simulink model "sampleModel1796"  (R2023a)
settings: Solver=VariableStepAuto  StartTime=0.0  StopTime=10.0  RelTol=1e-3
libraries: hdlsllib x7, simulink x1
settings Model: Creator=user1  LastModifiedBy=user1

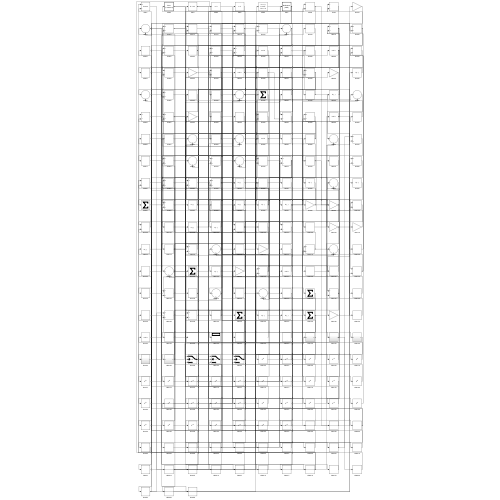
[thumbnail: Simulink's stored preview of the top-level diagram]
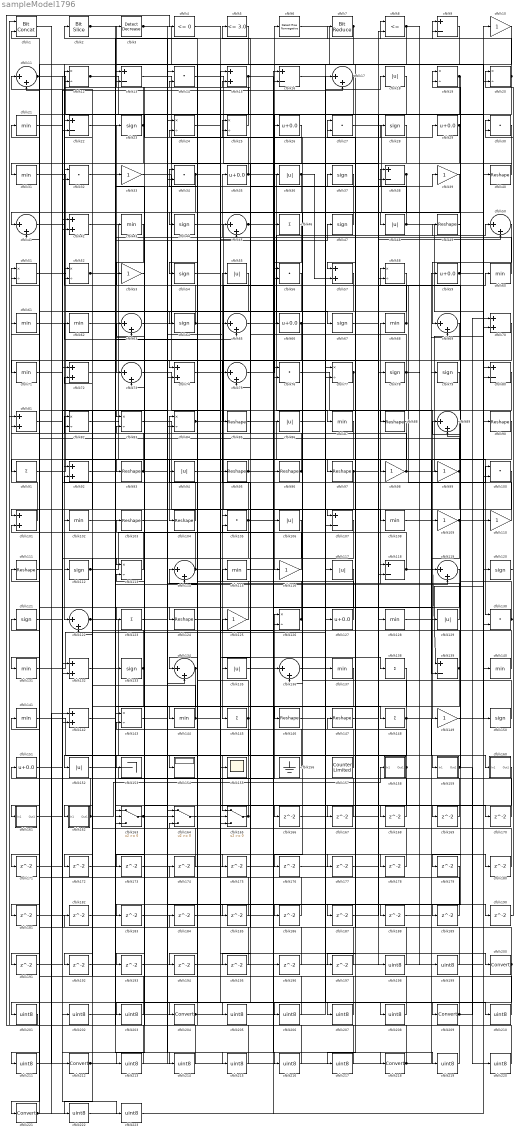
== system sampleModel1796 ==
  cfblk1 : hdlsllib/Logic and Bit Operations/Bit Concat  numInputs=2
  cfblk{10,33,39,53,98..99,109..110,116,125,149} (11 alike) : Gain
  cfblk{14,27,30,32,34,56,76,100,105,130} (10 alike) : DotProduct  OutDataTypeStr=Inherit: Inherit via internal rule
  cfblk{15,42,57,70,72,74,81,92,101,132,142} (11 alike) : Sum
  cfblk{21,31,43,60..62,68,71,87,102,108,115,128,131,137,140..141,144} (18 alike) : MinMax
  cfblk{40,49,85,88,90,93,95..97,103..104,111,124,146..147} (15 alike) : Reshape
  cfblk{18,36,48,55,86,94,106,117,129,135,152} (11 alike) : Abs  SaturateOnIntegerOverflow=off
  cfblk{9,13,16,22,38,80,107,118,139} (9 alike) : Sum  Inputs=+-
  cfblk{11,17,41,45,50,63,65,69,73,75,89,114,119,122,134,136} (16 alike) : Sum  Inputs=|++
  cfblk{23,28,37,44,47,54,64,67,78..79,112,120..121,133,150} (15 alike) : Signum
  cfblk{12,19..20,24..25,51..52,58,77,82..84,113,126,143} (15 alike) : Product  Inputs=*/  RndMeth=Zero  SaturateOnIntegerOverflow=on
  cfblk{46,91,123,138,145,148} (6 alike) : Sum  Inputs=+
  cfblk{26,29,35,59,66,127,151} (7 alike) : Bias  Bias=0.0  SaturateOnIntegerOverflow=off
  cfblk153 : Terminator
  cfblk154 : Display
  cfblk155 : Scope
  cfblk156 : Ground
  cfblk157 : hdlsllib/Sources/Counter Limited  uplimit=7  tsamp=-1
  cfblk158 : Subsystem
      settings: LibrarySourceBlock=|
      | hdlsllib/Ports &
      | Subsystems/Subsystem
  cfblk159 : Subsystem
      settings: LibrarySourceBlock=|
      | hdlsllib/Ports &
      | Subsystems/Subsystem
  cfblk160 : Subsystem
      settings: LibrarySourceBlock=|
      | hdlsllib/Ports &
      | Subsystems/Subsystem
  cfblk161 : Subsystem
      settings: LibrarySourceBlock=|
      | hdlsllib/Ports &
      | Subsystems/Subsystem
  cfblk162 : Subsystem
      settings: LibrarySourceBlock=|
      | hdlsllib/Ports &
      | Subsystems/Subsystem
  cfblk163 : Switch  SaturateOnIntegerOverflow=off  InputSameDT=off
  cfblk164 : Switch  SaturateOnIntegerOverflow=off  InputSameDT=off
  cfblk165 : Switch  SaturateOnIntegerOverflow=off  InputSameDT=off
  cfblk{166..197} (32 alike) : Delay  SampleTime=1
  cfblk{198..199,201..203,205..208,210..211,213..217,219..220,222..223} (20 alike) : DataTypeConversion  OutDataTypeStr=uint8  SaturateOnIntegerOverflow=off  RndMeth=Floor
  cfblk2 : hdlsllib/Logic and Bit Operations/Bit Slice  lidx=7  ridx=0
  cfblk{200,204,209,212,218,221} (6 alike) : DataTypeConversion  SaturateOnIntegerOverflow=off  RndMeth=Floor
  cfblk3 : simulink/Logic and Bit Operations/Detect Decrease  vinit=0.0  OutDataTypeStr=boolean
      settings: LibrarySourceBlock=|
      | hdlsllib/Logic and Bit
      | Operations/Detect
      | Decrease
  cfblk4 : hdlsllib/Logic and Bit Operations/Compare To Zero  relop=<=  OutDataTypeStr=boolean
  cfblk5 : hdlsllib/Logic and Bit Operations/Compare To Constant  relop=<=  const=3.0  OutDataTypeStr=boolean
  cfblk6 : hdlsllib/Logic and Bit Operations/Detect Rise Nonnegative  vinit=0  OutDataTypeStr=boolean
  cfblk7 : hdlsllib/Logic and Bit Operations/Bit Reduce  mode=AND
  cfblk8 : RelationalOperator  Operator=<=  OutDataTypeStr=boolean  InputSameDT=off
  wires:
  cfblk129/1 -> cfblk68/1
  cfblk63/1 -> cfblk27/1
  cfblk10/1 -> cfblk122/1
  cfblk122/1 -> cfblk154/1, cfblk47/1
  cfblk91/1 -> cfblk98/1
  cfblk68/1 -> cfblk12/1, cfblk64/1
  cfblk117/1 -> cfblk204/1
  cfblk60/1 -> cfblk35/1
  cfblk25/1 -> cfblk3/1
  cfblk152/1 -> cfblk126/1
  cfblk4/1 -> cfblk200/1
  cfblk31/1 -> cfblk93/1
  cfblk74/1 -> cfblk145/1
  cfblk87/1 -> cfblk104/1
  cfblk42/1 -> cfblk149/1
  cfblk46/1 -> cfblk116/1
  cfblk94/1 -> cfblk105/1
  cfblk64/1 -> cfblk23/1, cfblk138/1
  cfblk43/1 -> cfblk73/1
  cfblk162/1(Out1) -> cfblk158/1(In1), cfblk141/1
  cfblk66/1 -> cfblk123/1, cfblk49/1
  cfblk133/1 -> cfblk22/1, cfblk192/1
  cfblk113/1 -> cfblk103/1
  cfblk75/1 -> cfblk6/1
  cfblk56/1 -> cfblk112/1
  cfblk26/1 -> cfblk124/1
  cfblk65/1 -> cfblk50/1
  cfblk29/1 -> cfblk31/1, cfblk75/2, cfblk189/1
  cfblk17/1 -> cfblk96/1, cfblk153/1
  cfblk116/1 -> cfblk33/1
  cfblk85/1 -> cfblk130/1
  cfblk139/1 -> cfblk11/1, cfblk187/1
  cfblk130/1 -> cfblk30/1, cfblk56/2
  cfblk118/1 -> cfblk139/1, cfblk82/1
  cfblk41/1 -> cfblk52/1
  cfblk44/1 -> cfblk107/1
  cfblk47/1 -> cfblk41/1
  cfblk105/1 -> cfblk55/1, cfblk132/2, cfblk167/1
  cfblk23/1 -> cfblk101/1, cfblk12/2
  cfblk69/1 -> cfblk92/1
  cfblk28/1 -> cfblk135/1
  cfblk52/1 -> cfblk128/1, cfblk75/1
  cfblk156/1 -> cfblk115/1
  cfblk140/1 -> cfblk95/1
  cfblk83/1 -> cfblk108/1
  cfblk50/1 -> cfblk69/1
  cfblk145/1 -> cfblk152/1, cfblk114/1
  cfblk90/1 -> cfblk97/1
  cfblk34/1 -> cfblk48/1, cfblk173/1
  cfblk35/1 -> cfblk87/1, cfblk13/2
  cfblk3/1 -> cfblk137/1, cfblk186/1
  cfblk165/1 -> cfblk34/1, cfblk14/2
  cfblk134/1 -> cfblk114/2, cfblk222/1
  cfblk104/1 -> cfblk84/1
  cfblk148/1 -> cfblk165/1, cfblk160/1(In1), cfblk25/1, cfblk217/1
  cfblk7/1 -> cfblk144/1, cfblk11/2
  cfblk95/1 -> cfblk86/1, cfblk91/1
  cfblk136/1 -> cfblk18/1
  cfblk13/1 -> cfblk45/1
  cfblk125/1 -> cfblk2/1
  cfblk54/1 -> cfblk36/1
  cfblk51/1 -> cfblk67/1
  cfblk157/1 -> cfblk63/1
  cfblk30/1 -> cfblk134/1
  cfblk149/1 -> cfblk90/1
  cfblk114/1 -> cfblk29/1, cfblk51/2
  cfblk109/1 -> cfblk10/1, cfblk139/2
  cfblk84/1 -> cfblk26/1, cfblk170/1
  cfblk57/1 -> cfblk163/2
  cfblk78/1 -> cfblk43/1, cfblk99/1, cfblk146/1
  cfblk16/1 -> cfblk209/1
  cfblk98/1 -> cfblk40/1, cfblk25/2
  cfblk76/1 -> cfblk109/1
  cfblk14/1 -> cfblk78/1
  cfblk77/1 -> cfblk102/1, cfblk136/2, cfblk142/2
  cfblk49/1 -> cfblk19/1
  cfblk80/1 -> cfblk221/1
  cfblk36/1 -> cfblk57/2, cfblk193/1
  cfblk142/1 -> cfblk39/1
  cfblk27/1 -> cfblk150/1
  cfblk101/1 -> cfblk51/1
  cfblk20/1 -> cfblk107/2, cfblk9/2, cfblk191/1
  cfblk97/1 -> cfblk60/1, cfblk50/2, cfblk195/1
  cfblk8/1 -> cfblk197/1, cfblk199/1
  cfblk33/1 -> cfblk76/2
  cfblk92/1 -> cfblk133/1
  cfblk19/1 -> cfblk34/2, cfblk54/1, cfblk89/2
  cfblk121/1 -> cfblk17/2
  cfblk108/1 -> cfblk79/1
  cfblk40/1 -> cfblk32/1
  cfblk151/1 -> cfblk100/1
  cfblk22/1 -> cfblk148/1
  cfblk55/1 -> cfblk161/1(In1)
  cfblk82/1 -> cfblk119/1
  cfblk103/1 -> cfblk8/1
  cfblk110/1 -> cfblk58/1
  cfblk6/1 -> cfblk120/1
  cfblk73/1 -> cfblk155/1
  cfblk126/1 -> cfblk53/1, cfblk83/2
  cfblk141/1 -> cfblk159/1(In1)
  cfblk12/1 -> cfblk56/1, cfblk20/2
  cfblk2/1 -> cfblk119/2, cfblk208/1
  cfblk99/1 -> cfblk131/1, cfblk61/1, cfblk205/1
  cfblk61/1 -> cfblk74/1
  cfblk164/1 -> cfblk126/2
  cfblk48/1 -> cfblk70/2, cfblk5/1
  cfblk59/1 -> cfblk100/2, cfblk19/2
  cfblk93/1 -> cfblk21/1, cfblk7/1
  cfblk146/1 -> cfblk28/1
  cfblk32/1 -> cfblk164/2
  cfblk115/1 -> cfblk38/1
  cfblk143/1 -> cfblk218/1
  cfblk53/1 -> cfblk73/2
  cfblk62/1 -> cfblk9/1
  cfblk144/1 -> cfblk72/2, cfblk190/1
  cfblk11/1 -> cfblk72/1, cfblk140/1
  cfblk38/1 -> cfblk57/1, cfblk176/1
  cfblk79/1 -> cfblk88/1
  cfblk150/1 -> cfblk85/1
  cfblk5/1 -> cfblk44/1
  cfblk1/1 -> cfblk212/1
  cfblk128/1 -> cfblk110/1
  cfblk158/1(Out1) -> cfblk37/1, cfblk183/1
  cfblk21/1 -> cfblk84/2
  cfblk112/1 -> cfblk66/1, cfblk65/2
  cfblk96/1 -> cfblk15/2, cfblk82/2
  cfblk131/1 -> cfblk77/2
  cfblk9/1 -> cfblk71/1
  cfblk123/1 -> cfblk65/1
  cfblk132/1 -> cfblk63/2
  cfblk58/1 -> cfblk113/1
  cfblk159/1(Out1) -> cfblk89/1, cfblk220/1
  cfblk106/1 -> cfblk162/1(In1)
  cfblk127/1 -> cfblk62/1
  cfblk120/1 -> cfblk20/1
  cfblk15/1 -> cfblk42/2, cfblk168/1
  cfblk18/1 -> cfblk38/2
  cfblk39/1 -> cfblk83/1
  cfblk161/1(Out1) -> cfblk32/2
  cfblk163/1 -> cfblk118/1, cfblk188/1
  cfblk45/1 -> cfblk129/1, cfblk210/1
  cfblk88/1 -> cfblk166/1
  cfblk166/1 -> cfblk8/2
  cfblk167/1 -> cfblk113/2
  cfblk168/1 -> cfblk122/2
  cfblk124/1 -> cfblk169/1
  cfblk169/1 -> cfblk15/1
  cfblk170/1 -> cfblk42/1
  cfblk70/1 -> cfblk171/1
  cfblk171/1 -> cfblk22/2
  cfblk107/1 -> cfblk172/1
  cfblk172/1 -> cfblk58/2
  cfblk173/1 -> cfblk134/2
  cfblk174/1 -> cfblk14/1
  cfblk102/1 -> cfblk175/1
  cfblk175/1 -> cfblk17/1
  cfblk176/1 -> cfblk77/1
  cfblk72/1 -> cfblk177/1
  cfblk177/1 -> cfblk27/2
  cfblk86/1 -> cfblk178/1
  cfblk178/1 -> cfblk92/2
  cfblk100/1 -> cfblk179/1
  cfblk67/1 -> cfblk180/1
  cfblk180/1 -> cfblk165/2
  cfblk119/1 -> cfblk181/1
  cfblk181/1 -> cfblk45/2
  cfblk182/1 -> cfblk163/3
  cfblk183/1 -> cfblk136/1
  cfblk184/1 -> cfblk165/3
  cfblk89/1 -> cfblk185/1
  cfblk185/1 -> cfblk163/1
  cfblk186/1 -> cfblk41/2
  cfblk187/1 -> cfblk118/2
  cfblk188/1 -> cfblk69/2
  cfblk189/1 -> cfblk13/1
  cfblk190/1 -> cfblk30/2
  cfblk193/1 -> cfblk76/1
  cfblk138/1 -> cfblk194/1
  cfblk194/1 -> cfblk130/2
  cfblk195/1 -> cfblk132/1
  cfblk196/1 -> cfblk105/2
  cfblk197/1 -> cfblk52/2
  cfblk147/1 -> cfblk198/1
  cfblk198/1 -> cfblk94/1
  cfblk199/1 -> cfblk147/1
  cfblk200/1 -> cfblk125/1, cfblk151/1, cfblk211/1
  cfblk37/1 -> cfblk201/1
  cfblk201/1 -> cfblk4/1
  cfblk111/1 -> cfblk202/1
  cfblk202/1 -> cfblk106/1
  cfblk137/1 -> cfblk203/1
  cfblk203/1 -> cfblk111/1
  cfblk204/1 -> cfblk174/1, cfblk127/1
  cfblk205/1 -> cfblk117/1
  cfblk24/1 -> cfblk206/1
  cfblk206/1 -> cfblk182/1
  cfblk160/1(Out1) -> cfblk207/1
  cfblk207/1 -> cfblk24/1
  cfblk208/1 -> cfblk24/2
  cfblk209/1 -> cfblk101/2, cfblk70/1
  cfblk210/1 -> cfblk16/1
  cfblk211/1 -> cfblk16/2
  cfblk212/1 -> cfblk74/2, cfblk59/1, cfblk46/1
  cfblk179/1 -> cfblk213/1
  cfblk213/1 -> cfblk1/1
  cfblk192/1 -> cfblk214/1
  cfblk214/1 -> cfblk1/2
  cfblk81/1 -> cfblk215/1
  cfblk215/1 -> cfblk164/1
  cfblk71/1 -> cfblk216/1
  cfblk216/1 -> cfblk81/1
  cfblk217/1 -> cfblk81/2
  cfblk218/1 -> cfblk184/1, cfblk164/3
  cfblk135/1 -> cfblk219/1
  cfblk219/1 -> cfblk143/1
  cfblk220/1 -> cfblk143/2
  cfblk221/1 -> cfblk196/1, cfblk142/1, cfblk121/1
  cfblk222/1 -> cfblk80/1
  cfblk191/1 -> cfblk223/1
  cfblk223/1 -> cfblk80/2

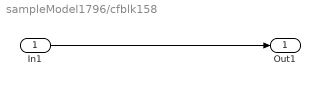
== system sampleModel1796/cfblk158 ==
  In1 : Inport
  Out1 : Outport
  wires:
  In1/1 -> Out1/1

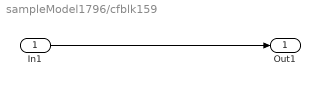
== system sampleModel1796/cfblk159 ==
  In1 : Inport
  Out1 : Outport
  wires:
  In1/1 -> Out1/1

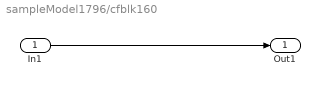
== system sampleModel1796/cfblk160 ==
  In1 : Inport
  Out1 : Outport
  wires:
  In1/1 -> Out1/1

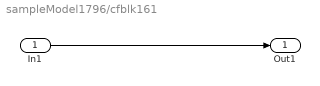
== system sampleModel1796/cfblk161 ==
  In1 : Inport
  Out1 : Outport
  wires:
  In1/1 -> Out1/1

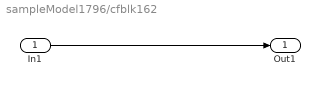
== system sampleModel1796/cfblk162 ==
  In1 : Inport
  Out1 : Outport
  wires:
  In1/1 -> Out1/1
